simulink model "IP_DLQ_VAR"  (R2022b)
settings: Solver=VariableStepAuto  StartTime=0.0  StopTime=t_sim  RelTol=1e-3
undefined symbols (not defined in the file): b1, b2, deltaT, DiscIntNeverNeededParam, etag, etam, g, Kgi, KliftS, km, kt, Lb, liftFun, Lp, mb, mp, Rm
libraries: simulink x1
settings Model: Creator=vince  LastModifiedBy=vince

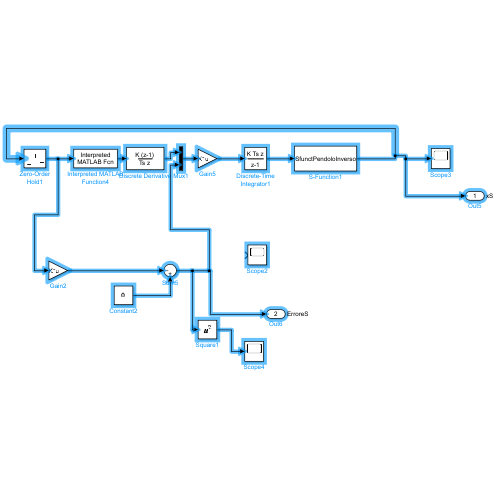
[thumbnail: Simulink's stored preview of the top-level diagram]
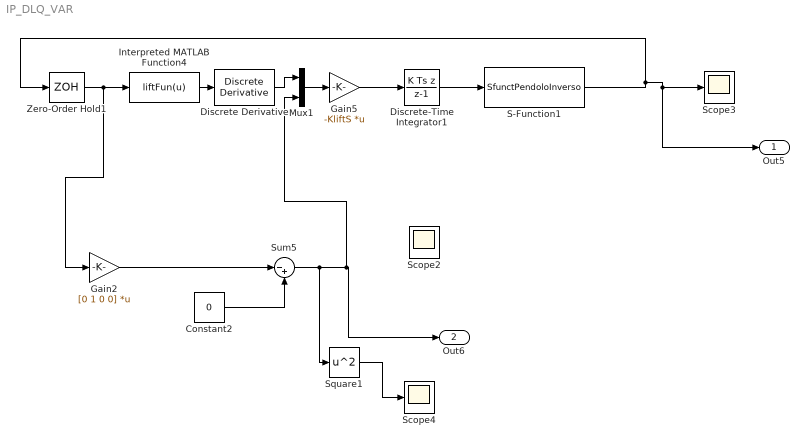
== system IP_DLQ_VAR ==
  Constant2 : Constant  Value=0
  Discrete Derivative : simulink/Discrete/Discrete Derivative  gainval=1  ICPrevScaledInput=0.0  OutMin=[]  OutMax=[]  OutDataType=fixdt(1, 16)  OutScaling=2^-10  DoSatur=off
  Discrete-Time Integrator1 : DiscreteIntegrator  IntegratorMethod=Integration: Backward Euler  SampleTime=deltaT  ICPrevOutput=DiscIntNeverNeededParam  ICPrevScaledInput=DiscIntNeverNeededParam
  Gain2 : Gain  Gain=[0 1 0 0]  Multiplication=Matrix(K*u)
  Gain5 : Gain  Gain=-KliftS  Multiplication=Matrix(K*u)
  Interpreted MATLAB Function4 : MATLABFcn  MATLABFcn=liftFun(u)
  Mux1 : Mux  Inputs=2
  S-Function1 : S-Function  FunctionName=SfunctPendoloInverso  Parameters=[0;0;0;0],mb,mp,Lb,Lp,b1,b2,g,Rm,kt,km,Kgi,etag,etam  SFunctionDeploymentMode=off  EnableBusSupport=off
  Scope2 : Scope
  Scope3 : Scope
  Scope4 : Scope
  Square1 : Math  Operator=square
  Sum5 : Sum  Inputs=|-+
  Zero-Order Hold1 : ZeroOrderHold  SampleTime=deltaT
  Out5 : Outport  SignalName=xS
  Out6 : Outport  Port=2  SignalName=ErroreS
  wires:
  Gain5/1 -> Discrete-Time Integrator1/1
  Discrete-Time Integrator1/1 -> S-Function1/1
  Sum5/1 -> Square1/1, Mux1/2, Out6/1
  Square1/1 -> Scope4/1
  Constant2/1 -> Sum5/2
  Interpreted MATLAB Function4/1 -> Discrete Derivative/1
  Discrete Derivative/1 -> Mux1/1
  Mux1/1 -> Gain5/1
  S-Function1/1 -> Out5/1, Scope3/1, Zero-Order Hold1/1
  Zero-Order Hold1/1 -> Gain2/1, Interpreted MATLAB Function4/1
  Gain2/1 -> Sum5/1
